simulink model "ueb1_1c"  (R2013a)
settings: Solver=ode4  StartTime=0.0  StopTime=60.0  FixedStep=h  RelTol=1e-3
values from neighbouring files (symbols this model uses):
  A = [-alpha 1;-2*beta*x(1)*x(2)-1 beta*(1-(x(1))^2)]    [aufg32d.m]    (also in wok.m = [0,1;-om0^2,-2*dvek(i)*om0])
undefined symbols (not defined in the file or in its folder): B, C, D
settings Model: Creator=isyssim2  LastModifiedBy=isyssim2

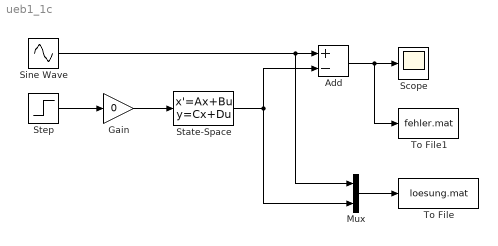
== system ueb1_1c ==
  Add : Sum  Inputs=+-
  Gain : Gain  Gain=0
  Mux : Mux  Inputs=2
  Scope : Scope
  Sine Wave : Sin  Amplitude=2*sqrt(2)  Frequency=0.5  Phase=-pi/4  SampleTime=0
  State-Space : StateSpace  A=A  B=B  C=C  D=D
  Step : Step  SampleTime=0
  To File : ToFile  Filename=loesung.mat  SaveFormat=Timeseries
  To File1 : ToFile  Filename=fehler.mat
  wires:
  Step/1 -> Gain/1
  Gain/1 -> State-Space/1
  State-Space/1 -> Mux/2, Add/2
  Sine Wave/1 -> Mux/1, Add/1
  Add/1 -> To File1/1, Scope/1
  Mux/1 -> To File/1
